simulink model "SMCC_Example_TestBench"  (R2019a)
settings: Solver=VariableStepAuto  StartTime=0.0  StopTime=23  RelTol=1e-3
PostLoadFcn:
  | helperLFSetUp
values from neighbouring files (symbols this model uses):
  Cf = 25    [SMCC_Parameters.m]
  Cr = 44    [SMCC_Parameters.m]
  lr = 0.15    [SMCC_Parameters.m]
  m = 2    [SMCC_Parameters.m]
  tau = 0.3    [SMCC_Parameters.m]
  Ts = 0.01    [SMCC_Parameters.m]
  v_set = 1.5    [SMCC_Parameters.m]
  Waypoints = [2.3 -0.0300000000000002 0 ... (first row only)    [SMCC_Parameters.m]
undefined symbols (not defined in the file or in its folder): driving, paramLS
libraries: drivingscenarioandsensors x2, autolibshared x1
settings Model: PauseTimes=7  Creator=The MathWorks, Inc.  LastModifiedBy=allenkim
settings DataIOCC: ReturnWorkspaceOutputs=off
settings DebuggingCC: ParameterPrecisionLossMsg=none  PregeneratedLibrarySubsystemCodeDiagnostic=none  ArithmeticOperatorsInVariantConditions=warning
settings HardwareCC: ProdLongLongMode=on
settings SFSimCC: SimUseLocalCustomCode=off
settings RTWCC: GenerateReport=on  RTWUseLocalCustomCode=off  LaunchReport=on
settings ConfigComp: CovScope=ReferencedModels  CovIncludeTopModel=off  CovHtmlReporting=on

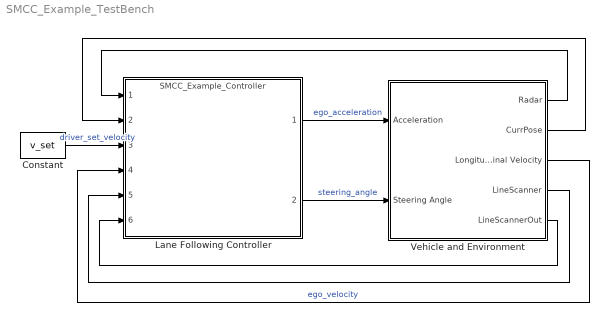
== system SMCC_Example_TestBench ==
  Constant : Constant  Value=v_set  SampleTime=Ts
  Lane Following Controller : ModelReference  ModelNameDialog=SMCC_Example_Controller.slx  SimulationMode=Normal  CodeInterface=Top model  ModelReferenceVersion=1.817
  Vehicle and Environment : Subsystem
  wires:
  Lane Following Controller/1 -> Vehicle and Environment/1(Acceleration)  "ego_acceleration"
  Lane Following Controller/2 -> Vehicle and Environment/2(Steering Angle)  "steering_angle"
  Constant/1 -> Lane Following Controller/3  "driver_set_velocity"
  Vehicle and Environment/3(Longitudinal Velocity) -> Lane Following Controller/4  "ego_velocity"
  Vehicle and Environment/4(LineScanner) -> Lane Following Controller/5
  Vehicle and Environment/1(Radar) -> Lane Following Controller/1
  Vehicle and Environment/2(CurrPose) -> Lane Following Controller/2
  Vehicle and Environment/5(LineScannerOut) -> Lane Following Controller/6

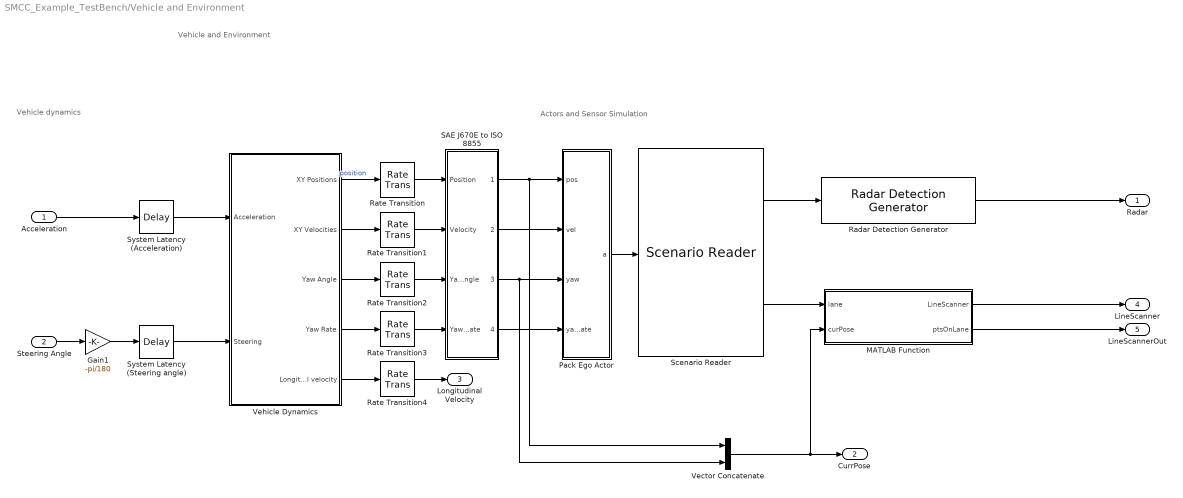
== system SMCC_Example_TestBench/Vehicle and Environment ==
  note: Vehicle dynamics
  note: Actors and Sensor Simulation
  note: Vehicle and Environment
  Acceleration : Inport  Unit=m/s^2
  Steering Angle : Inport  Port=2  Unit=rad
  Gain1 : Gain  Gain=-pi/180
  MATLAB Function : MATLAB Function  TreatAsAtomicUnit=on
  Pack Ego Actor : MATLAB Function  TreatAsAtomicUnit=on
  Radar Detection Generator : drivingscenarioandsensors/Radar Detection Generator  SensorIndex=2  UpdateInterval=Ts  SensorLocation=[ 0.3, 0 ]  Height=0.15  Yaw=0  Pitch=0  Roll=0  BusNameSource=Property  BusName=BusRadar  MaxNumDetectionsSource=Property  MaxNumDetections=10  DetectionCoordinates=Ego Cartesian  SimulateUsing=Interpreted execution  AzimuthResolution=4  ElevationResolution=10  RangeResolution=0.2  RangeRateResolution=0.5  AzimuthBiasFraction=0.1  ElevationBiasFraction=0.1  RangeBiasFraction=0.05  RangeRateBiasFraction=0.05  FieldOfView=[ 20, 5 ]  MaxRange=3  RangeRateLimits=[ -10, 10 ]  DetectionProbability=0.9  FalseAlarmRate=1e-6  ReferenceRange=1.5  ReferenceRCS=0  HasElevation=off  HasRangeRate=on  HasNoise=off  HasFalseAlarms=off  HasOcclusion=on  InitialSeedSource=Repeatable  InitialSeed=0  UsedSeed=driving.internal.SimulinkUtilities.seedManager(gcb)  ActorProfilesSource=MATLAB expression  ActorProfilesParameters=driving.internal.ActorProfilesRadarParameters  ActorProfilesExpression=actor_Profiles
      settings: SourceProductName=Automated Driving Toolbox  SourceProductBaseCode=DR
  Rate Transition{,1..4} (5 alike) : RateTransition  OutPortSampleTime=Ts
  SAE J670E to ISO 8855 : Subsystem
  Scenario Reader : drivingscenarioandsensors/Scenario Reader  ScenarioFileName=scenario_example_DoubleLane.mat  OutputCoordinateSystem=Vehicle coordinates  EgoVehicleSource=Input port  SampleTime=Ts  LaneBoundaryOutput=All lane boundaries  LaneBoundaryDistance=0:0.1:4  LaneBoundaryLocation=Inner edge of lane markings  BusNameSource=Auto  BusName2Source=Auto  SimulateUsing=Interpreted execution
      settings: SourceProductName=Automated Driving Toolbox
  System Latency (Acceleration) : TransportDelay  DelayTime=Ts
  System Latency (Steering angle) : TransportDelay  DelayTime=Ts
  Vector Concatenate : Concatenate
  Vehicle Dynamics : Subsystem  VariantControl=Variant2
  Radar : Outport
  CurrPose : Outport  Port=2
  Longitudinal Velocity : Outport  Port=3
  LineScanner : Outport  Port=4
  LineScannerOut : Outport  Port=5
  wires:
  Scenario Reader/1 -> Radar Detection Generator/1
  Vehicle Dynamics/2(XY Velocities) -> Rate Transition1/1
  Vehicle Dynamics/3(Yaw Angle) -> Rate Transition2/1
  Vehicle Dynamics/4(Yaw Rate) -> Rate Transition3/1
  Vehicle Dynamics/1(XY Positions) -> Rate Transition/1  "position"
  MATLAB Function/1(LineScanner) -> LineScanner/1
  Rate Transition4/1 -> Longitudinal Velocity/1
  Vehicle Dynamics/5(Longitudinal velocity) -> Rate Transition4/1
  Radar Detection Generator/1 -> Radar/1
  Pack Ego Actor/1(a) -> Scenario Reader/1
  Acceleration/1 -> System Latency (Acceleration)/1
  System Latency (Acceleration)/1 -> Vehicle Dynamics/1(Acceleration)
  System Latency (Steering angle)/1 -> Vehicle Dynamics/2(Steering)
  SAE J670E to ISO 8855/1(1) -> Vector Concatenate/1, Pack Ego Actor/1(pos)
  SAE J670E to ISO 8855/2(2) -> Pack Ego Actor/2(vel)
  SAE J670E to ISO 8855/3(3) -> Pack Ego Actor/3(yaw), Vector Concatenate/2
  SAE J670E to ISO 8855/4(4) -> Pack Ego Actor/4(yawRate)
  Rate Transition3/1 -> SAE J670E to ISO 8855/4(Yaw Rate)
  Rate Transition2/1 -> SAE J670E to ISO 8855/3(Yaw Angle)
  Rate Transition1/1 -> SAE J670E to ISO 8855/2(Velocity)
  Rate Transition/1 -> SAE J670E to ISO 8855/1(Position)
  Vector Concatenate/1 -> MATLAB Function/2(curPose), CurrPose/1
  Steering Angle/1 -> Gain1/1
  Gain1/1 -> System Latency (Steering angle)/1
  Scenario Reader/2 -> MATLAB Function/1(lane)
  MATLAB Function/2(ptsOnLane) -> LineScannerOut/1

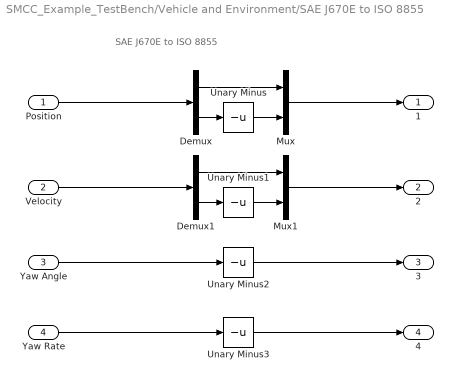
== system SMCC_Example_TestBench/Vehicle and Environment/SAE J670E to ISO 8855 ==
  note: SAE J670E to ISO 8855
  Position : Inport  Unit=m
  Velocity : Inport  Port=2  Unit=m/s
  Yaw Angle : Inport  Port=3  Unit=deg
  Yaw Rate : Inport  Port=4  Unit=deg/s
  Demux : Demux  Outputs=2
  Demux1 : Demux  Outputs=2
  Mux : Mux  Inputs=2
  Mux1 : Mux  Inputs=2
  Unary Minus{,1..3} (4 alike) : UnaryMinus
  1 : Outport
  2 : Outport  Port=2
  3 : Outport  Port=3
  4 : Outport  Port=4
  wires:
  Yaw Rate/1 -> Unary Minus3/1
  Yaw Angle/1 -> Unary Minus2/1
  Demux/1 -> Mux/1
  Demux/2 -> Unary Minus/1
  Unary Minus/1 -> Mux/2
  Unary Minus1/1 -> Mux1/2
  Demux1/2 -> Unary Minus1/1
  Demux1/1 -> Mux1/1
  Mux1/1 -> 2/1
  Mux/1 -> 1/1
  Position/1 -> Demux/1
  Velocity/1 -> Demux1/1
  Unary Minus2/1 -> 3/1
  Unary Minus3/1 -> 4/1

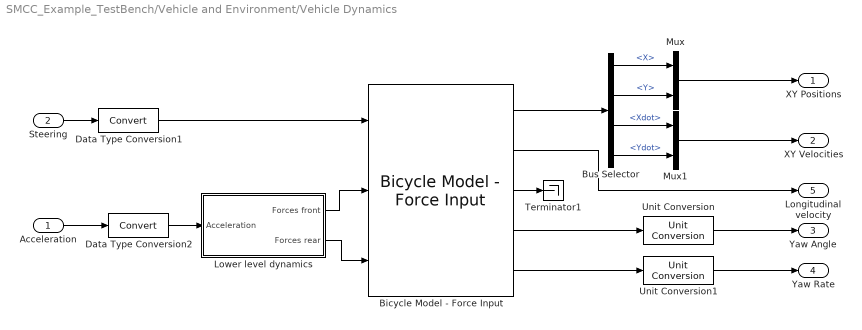
== system SMCC_Example_TestBench/Vehicle and Environment/Vehicle Dynamics ==
  Acceleration : Inport  Unit=m/s^2
  Steering : Inport  Port=2  Unit=rad
  Bicycle Model - Force Input : autolibshared/Bicycle Model - Force Input  trackMode=Single (bicycle)  inputMode=External longitudinal forces  frontSteerMode=on  rearSteerMode=off  windMode=off  muMode=off  extFMode=off  extMMode=off  aMode=3  NF=2  NR=2  m=m  a=lf  b=lr  h=0.05  X_o=x0_ego  xdot_o=v0_ego  CalphaMode=off  sigmaMode=on  w=[1.4,1.4]  Cy_f=Cf*100  Cy_r=Cr*100  sigma_f=.1  sigma_r=.1  alpha_f_brk=[-.1 .1]  Cy_f_data=[-9e3 9e3]  alpha_r_brk=[-.1 .1]  Cy_r_data=[-9e3 9e3]  Y_o=y0_ego  ydot_o=0  Izz=Iz  psi_o=yaw0_ego  r_o=0  Af=0  Cd=.3  Cl=.1  Cpm=.1  beta_w=[0:0.01:0.3]  Cs=[0:0.03:0.9]  Cym=[0:0.01:0.3]  Pabs=101325  Tair=273  g=9.81  mu=1  xdot_tol=.01  Fznom=5000  Fxtire_sat=1e6  Fytire_sat=1e6  longOff=0  latOff=0  vertOff=0
      settings: SourceProductName=Powertrain Blockset  SourceProductBaseCode=PW
  Bus Selector : BusSelector  OutputSignals=InertFrm.FrntAxl.Disp.X,InertFrm.FrntAxl.Disp.Y,InertFrm.FrntAxl.Vel.Xdot,InertFrm.FrntAxl.Vel.Ydot
  Data Type Conversion1 : DataTypeConversion
  Data Type Conversion2 : DataTypeConversion
  Lower level dynamics : Subsystem
  Mux : Mux  Inputs=2
  Mux1 : Mux  Inputs=2
  Terminator1 : Terminator
  Unit Conversion : UnitConversion  OutputType=Inherit: Inherit via back propagation
  Unit Conversion1 : UnitConversion  OutputType=Inherit: Inherit via back propagation
  XY Positions : Outport  Unit=m
  XY Velocities : Outport  Port=2  Unit=m/s
  Yaw Angle : Outport  Port=3  Unit=deg
  Yaw Rate : Outport  Port=4  Unit=degree/s
  Longitudinal velocity : Outport  Port=5
  wires:
  Lower level dynamics/2(Forces rear) -> Bicycle Model - Force Input/3
  Lower level dynamics/1(Forces front) -> Bicycle Model - Force Input/2
  Data Type Conversion2/1 -> Lower level dynamics/1(Acceleration)
  Data Type Conversion1/1 -> Bicycle Model - Force Input/1
  Acceleration/1 -> Data Type Conversion2/1
  Steering/1 -> Data Type Conversion1/1
  Bus Selector/1 -> Mux/1  "<X>"
  Unit Conversion/1 -> Yaw Angle/1
  Bicycle Model - Force Input/5 -> Unit Conversion1/1
  Bus Selector/4 -> Mux1/2  "<Ydot>"
  Bicycle Model - Force Input/4 -> Unit Conversion/1
  Bus Selector/2 -> Mux/2  "<Y>"
  Bicycle Model - Force Input/2 -> Longitudinal velocity/1
  Bus Selector/3 -> Mux1/1  "<Xdot>"
  Bicycle Model - Force Input/1 -> Bus Selector/1
  Bicycle Model - Force Input/3 -> Terminator1/1
  Mux/1 -> XY Positions/1
  Mux1/1 -> XY Velocities/1
  Unit Conversion1/1 -> Yaw Rate/1

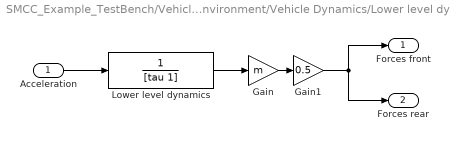
== system SMCC_Example_TestBench/Vehicle and Environment/Vehicle Dynamics/Lower level dynamics ==
  Acceleration : Inport
  Gain : Gain  Gain=m
  Gain1 : Gain  Gain=0.5
  Lower level dynamics : TransferFcn  Denominator=[tau 1]
  Forces front : Outport
  Forces rear : Outport  Port=2
  wires:
  Gain/1 -> Gain1/1
  Gain1/1 -> Forces front/1, Forces rear/1
  Acceleration/1 -> Lower level dynamics/1
  Lower level dynamics/1 -> Gain/1

== matlab function SMCC_Example_TestBench/Vehicle and Environment/MATLAB Function ==
  data: lane input; LineScanner output Bus: LaneSensor; paramLS parameter; Waypoints parameter; curPose input; ptsOnLane output
function [LineScanner,ptsOnLane] = fcn(lane,paramLS,Waypoints, curPose)

coder.extrinsic('fit','disp');

LaneBoundary.Curvature           = single(0);
LaneBoundary.CurvatureDerivative = single(0);
LaneBoundary.HeadingAngle        = single(0);
LaneBoundary.LateralOffset       = single(0);
LaneBoundary.Strength            = single(0);
sensorOut = zeros(128,4);
ptsOnLane = zeros(5,2);
ptOnLane = 0;

k = 0;
for i = 1:paramLS.numLineScanner
    pose = paramLS.LS(1).InstallPose(1:2);
    h    = paramLS.LS(1).InstallPose(3);
    srot = paramLS.LS(1).InstallPose(4:5);
    
    l = h/tan(srot(1)*pi/180);
    s = sqrt(h^2+l^2);
    
    for j = 1:lane.NumLaneBoundaries
        if ~isnan(lane.LaneBoundaries(j).Strength)
            % move lane pts to sensor coordinate
            lane_pts = lane.LaneBoundaries(j).Coordinates(:,1:2) - ones(length(lane.LaneBoundaries(j).Coordinates),1)*pose;
            theta    = srot(2)*pi/180;            
            lane_pts = ([cos(theta),sin(theta);-sin(theta),cos(theta)] * lane_pts')';
            
            if max(lane_pts(:,1)) < l || min(lane_pts(:,1)) > l, continue;  end
            if max(lane_pts(:,2)) < l || min(lane_pts(:,2)) > l, continue;  end
            lane_pts = lane_pts(lane_pts(:,1) < l+0.2 & lane_pts(:,1) > l-0.2 & abs(ptOnLane) <= s,:);
            if size(lane_pts,1) < 2, continue;end
            
            f = fit(lane_pts(:,1),lane_pts(:,2),'smoothingspline','SmoothingParam',0.07);
            ptOnLane = double(f(l));
            if abs(ptOnLane) <= s/2
                idx = floor((ptOnLane+s/2)/s*128);
                if idx == 0
                    idx = 1;
                end
                sensorOut(idx,i) = 200;
                k = k + 1;
                ptsOnLane(j,:) = ([cos(theta),-sin(theta);sin(theta),cos(theta)] * [l;ptOnLane])'+ pose;
            end
        end
    end
end


a = curPose;
b = Waypoints;
    
LineScanner.Left = LaneBoundary;
LineScanner.Right = LaneBoundary;

lpt = lane.LaneBoundaries(1).Coordinates(:,1:2);
rpt = lane.LaneBoundaries(2).Coordinates(:,1:2);

lheading = atan((lpt(2,2)-lpt(1,2))/(lpt(2,1)-lpt(1,1)));
rheading = atan((rpt(2,2)-rpt(1,2))/(rpt(2,1)-rpt(1,1)));

LineScanner.Left.HeadingAngle   = single(lheading);
LineScanner.Left.LateralOffset  = single(lpt(1,2));
LineScanner.Left.Strength       = single(lane.LaneBoundaries(1).Strength);
LineScanner.Right.HeadingAngle  = single(rheading);
LineScanner.Right.LateralOffset = single(rpt(1,2));
LineScanner.Right.Strength      = single(lane.LaneBoundaries(2).Strength);

== matlab function SMCC_Example_TestBench/Vehicle and Environment/Pack Ego Actor ==
  data: pos input; a output Bus: BusActors1Actors size=1; vel input; yaw input; yawRate input
function a = packEgo(pos,vel,yaw,yawRate)
% Pack ego information into a single ego actor bus
%
% Imoprtant note:
% Output is a bus of type BusActorsActors. This is the same bus used by the
% Scenario Reader to output an individual actor. If you change the
% output bus name of Scenario Reader change the output bus name here
% as well by clicking on 'Edit Data' in the menu above.

a = struct(...
    'ActorID',1,...
    'Position', [pos(1) pos(2) 0], ...
    'Velocity', [vel(1) vel(2) 0], ...
    'Roll', 0, ...
    'Pitch', 0, ...
    'Yaw', yaw, ...
    'AngularVelocity', [0 0 yawRate]);
